simulink library "NMCCPG_Library"  (R2016b)
settings: Solver=VariableStepAuto  StartTime=0.0  StopTime=10.0  RelTol=1e-3  EnableMultiTasking=on
undefined symbols (not defined in the file or in its folder): CPG_On, CPGPhaseCheckTs, CPGSaved, N_record, N_start, NoiseFs, Pc, Var_Fm, Var_L, Var_Vel
libraries: simulink x4, dspsigops x4
settings Model: Creator=brug  LastModifiedBy=tycho
settings DataIOCC: LimitDataPoints=on
settings OptimizationCC: LifeSpan=inf
settings DebuggingCC: AllowSymbolicDim=off  SFUnexpectedBacktrackingDiag=warning  SFNoUnconditionalDefaultTransitionDiag=warning  SFExecutionAtInitializationDiag=none
settings ModelReferenceCC: PropagateSignalLabelsOutOfModel=off
settings GRTTargetCC: TargetLangStandard=C89/C90 (ANSI)
settings ConfigComp: CovMetricSettings=dw  CovHtmlReporting=on  CovSaveCumulativeToWorkspaceVar=on  CovSaveSingleToWorkspaceVar=on  CovExternalEMLEnable=off

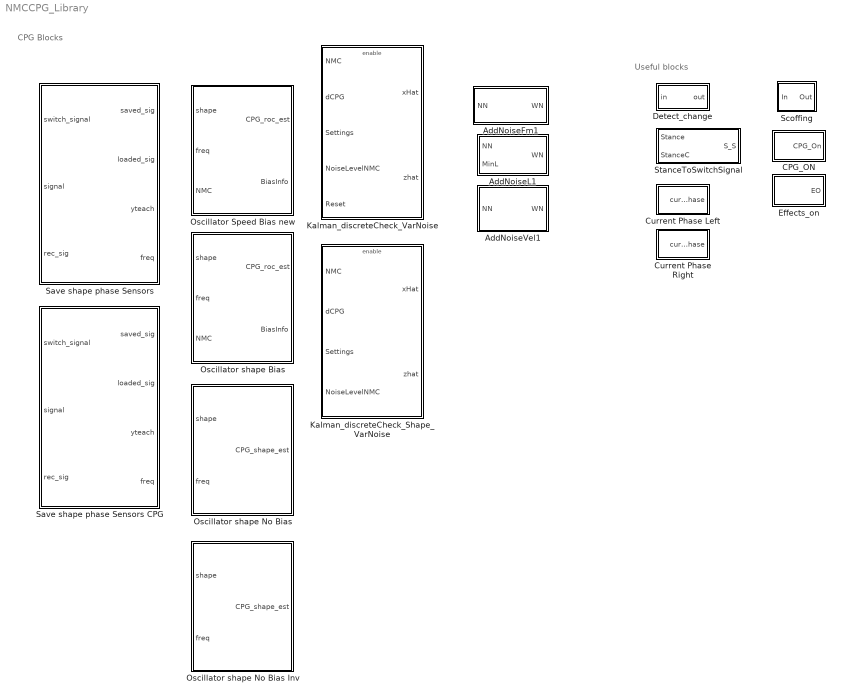
== system NMCCPG_Library ==
  note: CPG Blocks
  note: Useful blocks
  AddNoiseFm1 : Subsystem
  AddNoiseL1 : Subsystem
  AddNoiseVel1 : Subsystem
  CPG_ON : Subsystem
  Current Phase Left : Subsystem
  Current Phase Right : Subsystem
  Detect_change : Subsystem
  Effects_on : Subsystem
  Kalman_discreteCheck_Shape_VarNoise : Subsystem
      settings: MinAlgLoopOccurrences=on
  Kalman_discreteCheck_VarNoise : Subsystem
      settings: MinAlgLoopOccurrences=on
  "Oscillator Speed Bias new " : Subsystem
  Oscillator shape Bias : Subsystem
  Oscillator shape No Bias : Subsystem
  Oscillator shape No Bias Inv : Subsystem
  Save shape phase Sensors : Subsystem
  Save shape phase Sensors CPG : Subsystem
  Scoffing : Subsystem
  StanceToSwitchSignal : Subsystem

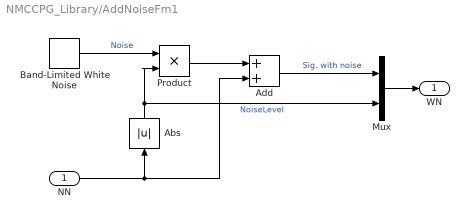
== system NMCCPG_Library/AddNoiseFm1 ==
  NN : Inport
  Abs : Abs
  Add : Sum
  Band-Limited White Noise : simulink/Sources/Band-Limited White Noise  Cov=[Var_Fm*(1/NoiseFs)]  Ts=(1/NoiseFs)  seed=[round(rand*10000)]
  Mux : Mux  Inputs=2
  Product : Product
  "WN " : Outport
  wires:
  Band-Limited White Noise/1 -> Product/1  "Noise"
  Product/1 -> Add/1
  NN/1 -> Abs/1, Add/2
  Add/1 -> Mux/1  "Sig. with noise"
  Mux/1 -> "WN "/1
  Abs/1 -> Product/2, Mux/2  "NoiseLevel"

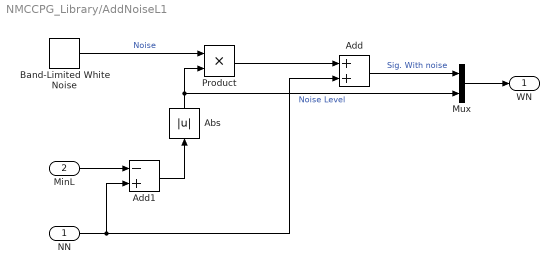
== system NMCCPG_Library/AddNoiseL1 ==
  NN : Inport
  MinL : Inport  Port=2
  Abs : Abs
  Add : Sum
  Add1 : Sum  Inputs=-+
  Band-Limited White Noise : simulink/Sources/Band-Limited White Noise  Cov=[Var_L*(1/NoiseFs)]  Ts=(1/NoiseFs)  seed=[round(rand*10000)]
  Mux : Mux  Inputs=2
  Product : Product
  "WN " : Outport
  wires:
  NN/1 -> Add1/2, Add/2
  Band-Limited White Noise/1 -> Product/1  "Noise"
  Product/1 -> Add/1
  Add1/1 -> Abs/1
  MinL/1 -> Add1/1
  Add/1 -> Mux/1  "Sig. With noise"
  Mux/1 -> "WN "/1
  Abs/1 -> Product/2, Mux/2  "Noise Level"

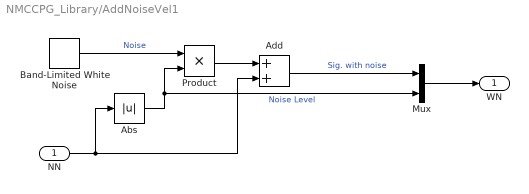
== system NMCCPG_Library/AddNoiseVel1 ==
  NN : Inport
  Abs : Abs
  Add : Sum
  Band-Limited White Noise : simulink/Sources/Band-Limited White Noise  Cov=[Var_Vel*(1/NoiseFs)]  Ts=(1/NoiseFs)  seed=[round(rand*10000)]
  Mux : Mux  Inputs=2
  Product : Product
  "WN " : Outport
  wires:
  NN/1 -> Add/2, Abs/1
  Abs/1 -> Mux/2, Product/2  "Noise Level"
  Band-Limited White Noise/1 -> Product/1  "Noise"
  Product/1 -> Add/1
  Mux/1 -> "WN "/1
  Add/1 -> Mux/1  "Sig. with noise"

== system NMCCPG_Library/CPG_ON ==
  Constant2 : Constant  Value=CPG_On
  Logical Operator : Logic  AllPortsSameDT=off  OutDataTypeStr=boolean
  CPG_On : Outport
  wires:
  [LR_saved_kept] -> Logical Operator/2
  Constant2/1 -> Logical Operator/1
  Logical Operator/1 -> CPG_On/1

== system NMCCPG_Library/Current Phase Left ==
  Sample and Hold3 : dspsigops/Sample and Hold  trig=Rising edge  initCond=0  latchinput=off
  cur_phase : Outport
  wires:
  Sample and Hold3/1 -> cur_phase/1
  [SwitchL] -> Sample and Hold3/Trigger, Sample and Hold3/1

== system NMCCPG_Library/Current Phase Right ==
  Sample and Hold3 : dspsigops/Sample and Hold  trig=Rising edge  initCond=0  latchinput=off
  cur_phase : Outport
  wires:
  [SwitchR] -> Sample and Hold3/1, Sample and Hold3/Trigger
  Sample and Hold3/1 -> cur_phase/1

== system NMCCPG_Library/Detect_change ==
  note: U(k)
  note: Edge
  in : Inport
  FixPt Relational Operator : RelationalOperator  Operator=~=  OutDataTypeStr=fixdt(0, 8)  ZeroCross=off  RndMeth=Nearest
  Memory : Memory
  "out " : Outport
  wires:
  Memory/1 -> FixPt Relational Operator/2  "U(k-1)"
  FixPt Relational Operator/1 -> "out "/1
  in/1 -> FixPt Relational Operator/1, Memory/1

== system NMCCPG_Library/Effects_on ==
  note: Used to turn on:
      | - Disturbances
      | - Noise on sensory signal
  Data Type Conversion : DataTypeConversion
  Transport Delay3 : TransportDelay  DelayTime=0.1
  EO : Outport
  wires:
  [LR_saved_kept] -> Data Type Conversion/1
  Transport Delay3/1 -> EO/1
  Data Type Conversion/1 -> Transport Delay3/1

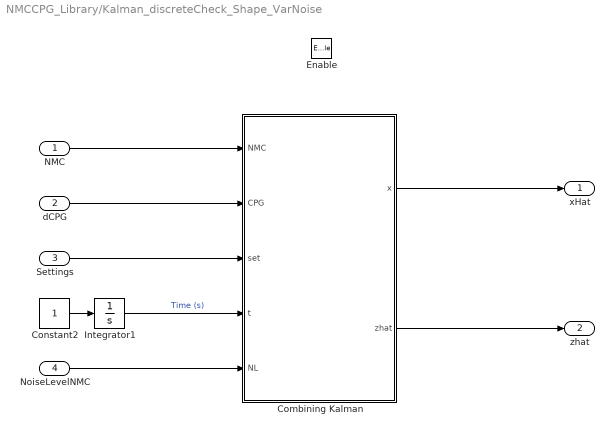
== system NMCCPG_Library/Kalman_discreteCheck_Shape_VarNoise ==
  NMC : Inport
  dCPG : Inport  Port=2
  Settings : Inport  Port=3
  NoiseLevelNMC : Inport  Port=4
  Enable : EnablePort  StatesWhenEnabling=reset
  Combining Kalman : MATLAB Function  SystemSampleTime=1E-3
      settings: MinAlgLoopOccurrences=on
  Constant2 : Constant
  Integrator1 : Integrator
  xHat : Outport
  zhat : Outport  Port=2
  wires:
  NoiseLevelNMC/1 -> Combining Kalman/5(NL)
  Combining Kalman/2(zhat) -> zhat/1
  Combining Kalman/1(x) -> xHat/1
  NMC/1 -> Combining Kalman/1(NMC)
  Settings/1 -> Combining Kalman/3(set)
  Constant2/1 -> Integrator1/1
  Integrator1/1 -> Combining Kalman/4(t)  "Time (s)"
  dCPG/1 -> Combining Kalman/2(CPG)

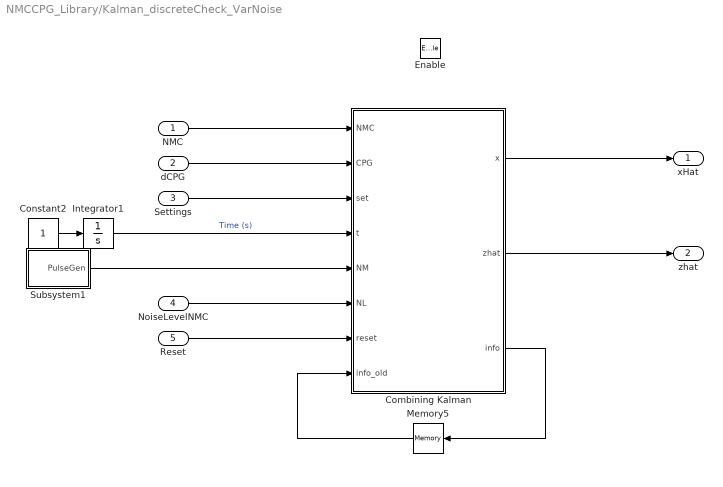
== system NMCCPG_Library/Kalman_discreteCheck_VarNoise ==
  NMC : Inport
  dCPG : Inport  Port=2
  Settings : Inport  Port=3
  NoiseLevelNMC : Inport  Port=4
  Reset : Inport  Port=5
  Enable : EnablePort  StatesWhenEnabling=reset
  Combining Kalman : MATLAB Function  TreatAsAtomicUnit=on  SystemSampleTime=1E-3
      settings: MinAlgLoopOccurrences=on
  Constant2 : Constant
  Integrator1 : Integrator
  Memory5 : Memory  X0=zeros(59,1)
  Subsystem1 : Subsystem
  xHat : Outport
  zhat : Outport  Port=2
  wires:
  Reset/1 -> Combining Kalman/7(reset)
  dCPG/1 -> Combining Kalman/2(CPG)
  Memory5/1 -> Combining Kalman/8(info_old)
  Combining Kalman/3(info) -> Memory5/1
  Integrator1/1 -> Combining Kalman/4(t)  "Time (s)"
  Constant2/1 -> Integrator1/1
  Subsystem1/1(PulseGen) -> Combining Kalman/5(NM)
  Settings/1 -> Combining Kalman/3(set)
  NMC/1 -> Combining Kalman/1(NMC)
  Combining Kalman/1(x) -> xHat/1
  Combining Kalman/2(zhat) -> zhat/1
  NoiseLevelNMC/1 -> Combining Kalman/6(NL)

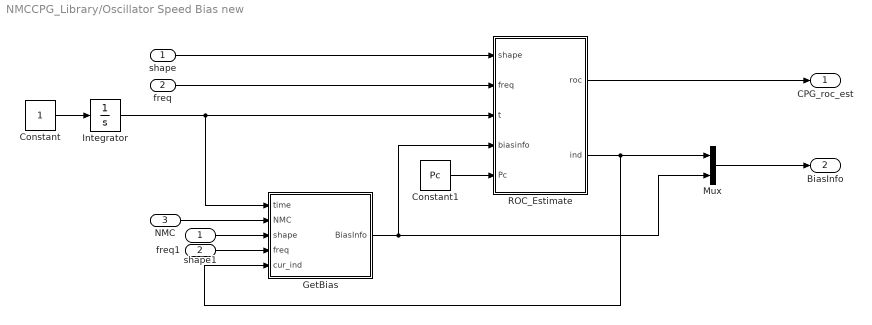
== system NMCCPG_Library/Oscillator Speed Bias new  ==
  shape : Inport
  freq : Inport  Port=2
  NMC : Inport  Port=3
  Constant : Constant
  Constant1 : Constant  Value=Pc
  GetBias : Subsystem
  Integrator : Integrator
  Mux : Mux  Inputs=2
  ROC_Estimate : MATLAB Function  TreatAsAtomicUnit=on
  freq1 : InportShadow  Port=2
  shape1 : InportShadow
  CPG_roc_est : Outport
  BiasInfo : Outport  Port=2
  wires:
  Constant1/1 -> ROC_Estimate/5(Pc)
  Mux/1 -> BiasInfo/1
  GetBias/1(BiasInfo) -> ROC_Estimate/4(biasinfo), Mux/2
  ROC_Estimate/2(ind) -> GetBias/5(cur_ind), Mux/1
  shape1/1 -> GetBias/3(shape)
  NMC/1 -> GetBias/2(NMC)
  Integrator/1 -> ROC_Estimate/3(t), GetBias/1(time)
  Constant/1 -> Integrator/1
  shape/1 -> ROC_Estimate/1(shape)
  ROC_Estimate/1(roc) -> CPG_roc_est/1
  freq/1 -> ROC_Estimate/2(freq)
  freq1/1 -> GetBias/4(freq)

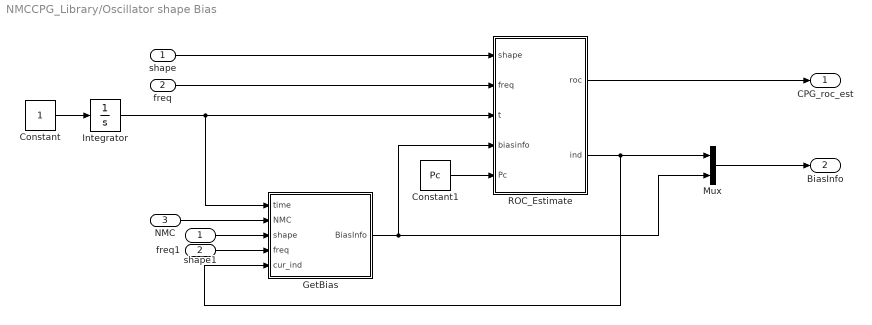
== system NMCCPG_Library/Oscillator shape Bias ==
  shape : Inport
  freq : Inport  Port=2
  NMC : Inport  Port=3
  Constant : Constant
  Constant1 : Constant  Value=Pc
  GetBias : Subsystem
  Integrator : Integrator
  Mux : Mux  Inputs=2
  ROC_Estimate : MATLAB Function  TreatAsAtomicUnit=on
  freq1 : InportShadow  Port=2
  shape1 : InportShadow
  CPG_roc_est : Outport
  BiasInfo : Outport  Port=2
  wires:
  freq1/1 -> GetBias/4(freq)
  freq/1 -> ROC_Estimate/2(freq)
  ROC_Estimate/1(roc) -> CPG_roc_est/1
  shape/1 -> ROC_Estimate/1(shape)
  Constant/1 -> Integrator/1
  Integrator/1 -> GetBias/1(time), ROC_Estimate/3(t)
  NMC/1 -> GetBias/2(NMC)
  shape1/1 -> GetBias/3(shape)
  ROC_Estimate/2(ind) -> Mux/1, GetBias/5(cur_ind)
  GetBias/1(BiasInfo) -> Mux/2, ROC_Estimate/4(biasinfo)
  Mux/1 -> BiasInfo/1
  Constant1/1 -> ROC_Estimate/5(Pc)

== system NMCCPG_Library/Oscillator shape No Bias ==
  shape : Inport
  freq : Inport  Port=2
  Constant : Constant
  Integrator : Integrator
  ROC_Estimate : MATLAB Function  TreatAsAtomicUnit=on  SystemSampleTime=1e-2
      settings: MinAlgLoopOccurrences=on
  CPG_shape_est : Outport
  wires:
  freq/1 -> ROC_Estimate/2(freq)
  ROC_Estimate/1(cpg_out) -> CPG_shape_est/1
  shape/1 -> ROC_Estimate/1(shape)
  Constant/1 -> Integrator/1
  Integrator/1 -> ROC_Estimate/3(t)

== system NMCCPG_Library/Oscillator shape No Bias Inv ==
  shape : Inport
  freq : Inport  Port=2
  Constant : Constant
  Integrator : Integrator
  ROC_Estimate : MATLAB Function  TreatAsAtomicUnit=on
      settings: MinAlgLoopOccurrences=on
  CPG_shape_est : Outport
  wires:
  Integrator/1 -> ROC_Estimate/3(t)
  Constant/1 -> Integrator/1
  shape/1 -> ROC_Estimate/1(shape)
  ROC_Estimate/1(cpg_out) -> CPG_shape_est/1
  freq/1 -> ROC_Estimate/2(freq)

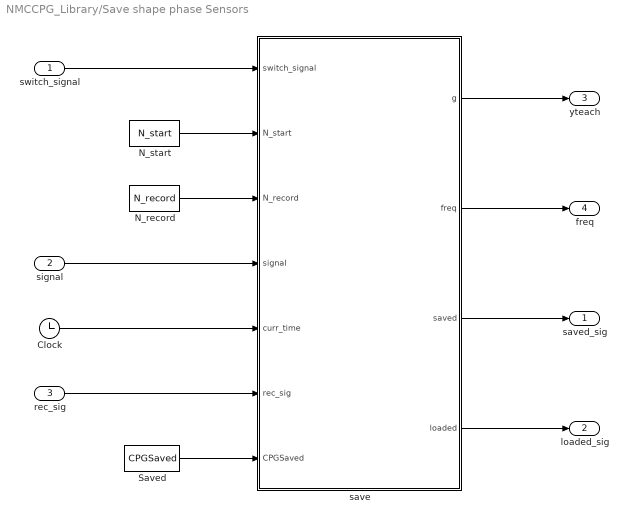
== system NMCCPG_Library/Save shape phase Sensors ==
  switch_signal : Inport
  signal : Inport  Port=2
  rec_sig : Inport  Port=3
  Clock : Clock
      settings: Decimation=1E6
  N_record : Constant  Value=N_record
  N_start : Constant  Value=N_start
  Saved : Constant  Value=CPGSaved
  save : Stateflow chart  TreatAsAtomicUnit=on
  saved_sig : Outport
  loaded_sig : Outport  Port=2
  yteach : Outport  Port=3
  freq : Outport  Port=4
  wires:
  Saved/1 -> save/7(CPGSaved)
  switch_signal/1 -> save/1(switch_signal)
  N_record/1 -> save/3(N_record)
  signal/1 -> save/4(signal)
  save/2(freq) -> freq/1
  N_start/1 -> save/2(N_start)
  save/1(g) -> yteach/1
  save/3(saved) -> saved_sig/1
  Clock/1 -> save/5(curr_time)
  rec_sig/1 -> save/6(rec_sig)
  save/4(loaded) -> loaded_sig/1

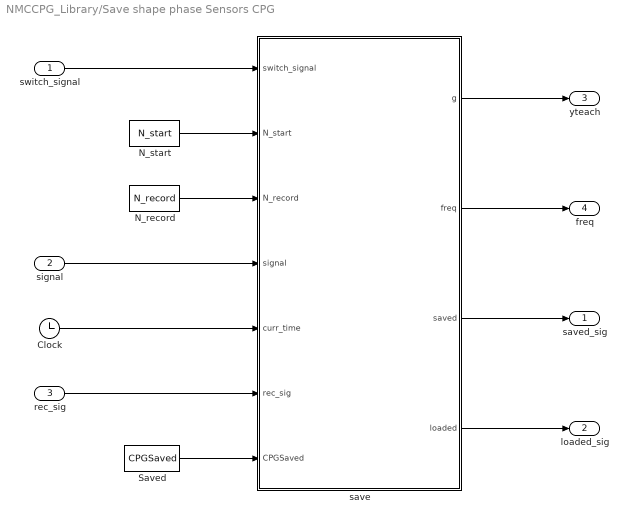
== system NMCCPG_Library/Save shape phase Sensors CPG ==
  switch_signal : Inport
  signal : Inport  Port=2
  rec_sig : Inport  Port=3
  Clock : Clock
      settings: Decimation=1E6
  N_record : Constant  Value=N_record
  N_start : Constant  Value=N_start
  Saved : Constant  Value=CPGSaved
  save : Stateflow chart  TreatAsAtomicUnit=on
  saved_sig : Outport
  loaded_sig : Outport  Port=2
  yteach : Outport  Port=3
  freq : Outport  Port=4
  wires:
  save/4(loaded) -> loaded_sig/1
  rec_sig/1 -> save/6(rec_sig)
  Clock/1 -> save/5(curr_time)
  save/3(saved) -> saved_sig/1
  save/1(g) -> yteach/1
  N_start/1 -> save/2(N_start)
  save/2(freq) -> freq/1
  signal/1 -> save/4(signal)
  N_record/1 -> save/3(N_record)
  switch_signal/1 -> save/1(switch_signal)
  Saved/1 -> save/7(CPGSaved)

== system NMCCPG_Library/Scoffing ==
  note: This Block keeps the swing phase active for 0.1s in case of scoffing
  In : Inport
  Compare To Zero : simulink/Logic and Bit Operations/Compare To Zero  relop=>  OutDataTypeStr=boolean
  Data Type Conversion : DataTypeConversion
  Logical Operator : Logic  Operator=OR  AllPortsSameDT=off  OutDataTypeStr=boolean
  Transport Delay : TransportDelay  DelayTime=0.1
  Out : Outport
  wires:
  Transport Delay/1 -> Compare To Zero/1
  In/1 -> Data Type Conversion/1, Logical Operator/2
  Logical Operator/1 -> Out/1
  Data Type Conversion/1 -> Transport Delay/1
  Compare To Zero/1 -> Logical Operator/1

== system NMCCPG_Library/StanceToSwitchSignal ==
  note: Change signal:
      | 1 - Stance
      | 2 - Swing
  Stance : Inport
  StanceC : Inport  Port=2
  MATLAB Function : MATLAB Function  TreatAsAtomicUnit=on
  S_S : Outport
  wires:
  StanceC/1 -> MATLAB Function/2(u2)
  MATLAB Function/1(y) -> S_S/1
  Stance/1 -> MATLAB Function/1(u1)

== system NMCCPG_Library/Kalman_discreteCheck_VarNoise/Subsystem1 ==
  Abs : Abs
  Add : Sum  Inputs=+-
  Memory : Memory
  Pulse Generator : DiscretePulseGenerator  PulseType=Time based  Period=(1/NoiseFs)*2  PulseWidth=50  SampleTime=-1
  PulseGen : Outport
  wires:
  Add/1 -> Abs/1
  Abs/1 -> PulseGen/1
  Memory/1 -> Add/2
  Pulse Generator/1 -> Add/1, Memory/1

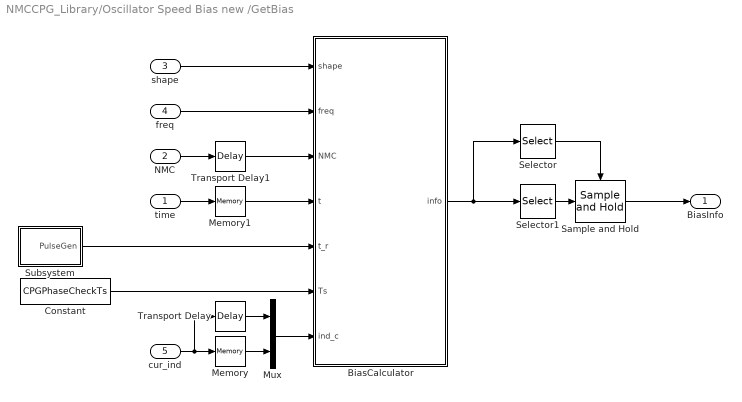
== system NMCCPG_Library/Oscillator Speed Bias new /GetBias ==
  time : Inport
  NMC : Inport  Port=2
  shape : Inport  Port=3
  freq : Inport  Port=4
  cur_ind : Inport  Port=5
  BiasCalculator : MATLAB Function  TreatAsAtomicUnit=on
  Constant : Constant  Value=CPGPhaseCheckTs
  Memory : Memory
  Memory1 : Memory
  Mux : Mux  Inputs=2
  Sample and Hold : dspsigops/Sample and Hold  trig=Rising edge  initCond=[]  latchinput=off
  Selector : Selector  InputPortWidth=4  IndexOptions=Index vector (dialog)  Indices=[1]  OutputSizes=1
  Selector1 : Selector  InputPortWidth=4  IndexOptions=Index vector (dialog)  Indices=[2:4]  OutputSizes=1
  Subsystem : Subsystem
  Transport Delay : TransportDelay  DelayTime=CPGPhaseCheckTs*0.5
  Transport Delay1 : TransportDelay  DelayTime=CPGPhaseCheckTs*0.5  InitialOutput=zeros(19,1)
  BiasInfo : Outport
  wires:
  Transport Delay1/1 -> BiasCalculator/3(NMC)
  Selector1/1 -> Sample and Hold/1
  Memory1/1 -> BiasCalculator/4(t)
  Mux/1 -> BiasCalculator/7(ind_c)
  Transport Delay/1 -> Mux/1
  Memory/1 -> Mux/2
  Selector/1 -> Sample and Hold/Trigger
  Sample and Hold/1 -> BiasInfo/1
  Subsystem/1(PulseGen) -> BiasCalculator/5(t_r)
  Constant/1 -> BiasCalculator/6(Ts)
  shape/1 -> BiasCalculator/1(shape)
  BiasCalculator/1(info) -> Selector/1, Selector1/1
  cur_ind/1 -> Memory/1, Transport Delay/1
  time/1 -> Memory1/1
  NMC/1 -> Transport Delay1/1
  freq/1 -> BiasCalculator/2(freq)

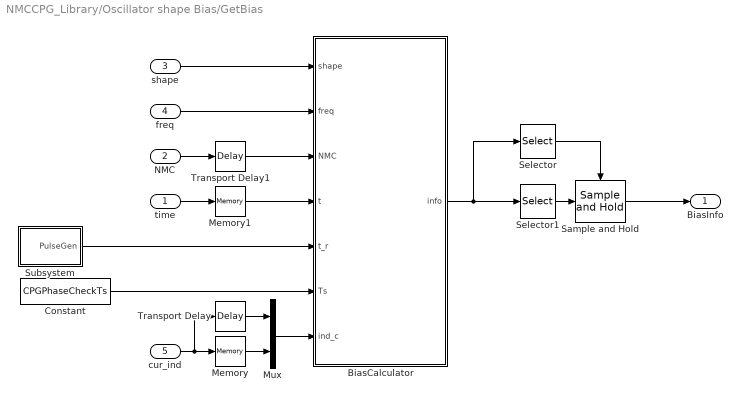
== system NMCCPG_Library/Oscillator shape Bias/GetBias ==
  time : Inport
  NMC : Inport  Port=2
  shape : Inport  Port=3
  freq : Inport  Port=4
  cur_ind : Inport  Port=5
  BiasCalculator : MATLAB Function  TreatAsAtomicUnit=on
  Constant : Constant  Value=CPGPhaseCheckTs
  Memory : Memory
  Memory1 : Memory
  Mux : Mux  Inputs=2
  Sample and Hold : dspsigops/Sample and Hold  trig=Rising edge  initCond=[]  latchinput=off
  Selector : Selector  InputPortWidth=4  IndexOptions=Index vector (dialog)  Indices=[1]  OutputSizes=1
  Selector1 : Selector  InputPortWidth=4  IndexOptions=Index vector (dialog)  Indices=[2:4]  OutputSizes=1
  Subsystem : Subsystem
  Transport Delay : TransportDelay  DelayTime=CPGPhaseCheckTs*0.5
  Transport Delay1 : TransportDelay  DelayTime=CPGPhaseCheckTs*0.5  InitialOutput=zeros(19,1)
  BiasInfo : Outport
  wires:
  freq/1 -> BiasCalculator/2(freq)
  NMC/1 -> Transport Delay1/1
  time/1 -> Memory1/1
  cur_ind/1 -> Transport Delay/1, Memory/1
  BiasCalculator/1(info) -> Selector1/1, Selector/1
  shape/1 -> BiasCalculator/1(shape)
  Constant/1 -> BiasCalculator/6(Ts)
  Subsystem/1(PulseGen) -> BiasCalculator/5(t_r)
  Sample and Hold/1 -> BiasInfo/1
  Selector/1 -> Sample and Hold/Trigger
  Memory/1 -> Mux/2
  Transport Delay/1 -> Mux/1
  Mux/1 -> BiasCalculator/7(ind_c)
  Memory1/1 -> BiasCalculator/4(t)
  Selector1/1 -> Sample and Hold/1
  Transport Delay1/1 -> BiasCalculator/3(NMC)

== system NMCCPG_Library/Oscillator Speed Bias new /GetBias/Subsystem ==
  note: PulseGen outputs a 1 every after every CPGPhaseCheckTs (s)
  Abs : Abs
  Add : Sum  Inputs=+-
  Memory : Memory
  Pulse Generator : DiscretePulseGenerator  PulseType=Time based  Period=CPGPhaseCheckTs*2  PulseWidth=50  SampleTime=-1
  PulseGen : Outport
  wires:
  Add/1 -> Abs/1
  Abs/1 -> PulseGen/1
  Memory/1 -> Add/2
  Pulse Generator/1 -> Add/1, Memory/1

== system NMCCPG_Library/Oscillator shape Bias/GetBias/Subsystem ==
  note: PulseGen outputs a 1 every after every CPGPhaseCheckTs (s)
  Abs : Abs
  Add : Sum  Inputs=+-
  Memory : Memory
  Pulse Generator : DiscretePulseGenerator  PulseType=Time based  Period=CPGPhaseCheckTs*2  PulseWidth=50  SampleTime=-1
  PulseGen : Outport
  wires:
  Pulse Generator/1 -> Memory/1, Add/1
  Memory/1 -> Add/2
  Abs/1 -> PulseGen/1
  Add/1 -> Abs/1

== matlab function NMCCPG_Library/Oscillator Speed Bias new /GetBias/BiasCalculator ==
  data: shape input; freq input; NMC input; t input; t_r input; Ts input; ind_c input; info output
function info  = fcn(shape,freq,NMC,t,t_r,Ts,ind_c)
%% SizeSettings
N = size(shape,2);
p_area = Ts*freq;

%% Initial conditions
if t < Ts
    info = [2+t;0;1;0];
else
    if t_r == 1 
        %% Estimated indices
        fg = ind_c(1);
        
        %% Setting size
        assert(fg<N*2) 
        assert(fg>-N*2);
        assert(p_area<10) 
        assert(p_area>-1);
        
        %% Max area
        area = round(fg)-round(p_area*N):round(fg)+round(p_area*N);
        area(area<1) = [];area(area>N) = [];
        
        %% Finding optimal index in shape
        cur = repmat(NMC,1,length(area));
        [~,ind2] = min(sum(abs(shape(:,area)-cur)));
        ind = ind2 + min(area) - 1;
        
        %% Calculating Bias
        bias = ind - fg;
        
        %% Setting output
        info = [1;bias;ind_c(2);t];
    else
        %% BiasCheck is only active if t_r == 1
        info = zeros(4,1);
    end
end

== matlab function NMCCPG_Library/Oscillator Speed Bias new /ROC_Estimate ==
  data: shape input; roc output; freq input; t input; biasinfo input; ind output; Pc input
function [roc,ind] = roc_est(shape,freq,t,biasinfo,Pc)
%% Pre-allocating
N = size(shape,2);
M = size(shape,1);
roc = zeros(M,1);

%% Estimating current indices in Shape
% Initial conditions
if t < 0.05 || biasinfo(2,1) == 1
    biasinfo = [0;1;0];
end

%% Calculating frequency
freq_n = (biasinfo(1,1)/(Pc*(N-1)))+freq;

%% Estimating current index in shape
ind = biasinfo(2,1) + (N-1)*(t-biasinfo(3,1))*freq_n;

%% Flooring and finding diff
ind_fl = floor(ind);
int_diff = ind-ind_fl;

%% Setting bounds
if ind > N
    ind = N;
    ind_fl = N;
end
assert(ind_fl<N+1) 
assert(ind_fl>0);

%% Calculating speed using 9 point diff and interpolating for extra accuracy
ind_l = zeros(1,10);
ind_l(1,:) = ind_fl-4:ind_fl+5;
if ind_l(1) >= 1 && ind_l(end) <= N
    x_int = zeros(M,9);
    x_int(:,:) = interp1(ind_l,shape(:,ind_l)',ind_l(1:end-1)+int_diff)';
    speed = sum(x_int.*repmat([1/280 -4/105 1/5 -4/5 0 4/5 -1/5 4/105 -1/280]*((N-1)*freq),size(x_int,1),1),2);
elseif ind_l(1) < 1
    x_int = zeros(M,5);
    x_int(:,:) = interp1(ind_l(5:end),shape(:,ind_l(5:end))',ind_l(5:end-1)+int_diff)';
    speed = sum(x_int.*repmat([-25/12 4 -3 4/3 -1/4]*((N-1)*freq),size(x_int,1),1),2);
elseif ind_l(6) < N
    x_int = zeros(M,5);
    x_int(:,:) = interp1(ind_l(1:6),shape(:,ind_l(1:6))',ind_l(1:5)+int_diff)';
    speed = sum(x_int.*repmat([1/4 -4/3 3 -4 25/12]*((N-1)*freq),size(x_int,1),1),2);
else
    speed = sum(shape(:,end-4:end).*repmat([1/4 -4/3 3 -4 25/12]*((N-1)*freq),size(shape(:,end-4:end),1),1),2);
end 

%% Output
roc(:,1) = speed;
end

== matlab function NMCCPG_Library/Oscillator shape Bias/GetBias/BiasCalculator ==
  data: shape input; freq input; NMC input; t input; t_r input; Ts input; ind_c input; info output
function info  = fcn(shape,freq,NMC,t,t_r,Ts,ind_c)
%% SizeSettings
N = size(shape,2);
p_area = Ts*freq;

%% Initial conditions
if t < Ts
    info = [2+t;0;1;0];
else
    if t_r == 1 
        %% Estimated indices
        fg = ind_c(1);
        
        %% Setting size
        assert(fg<N*2) 
        assert(fg>-N*2);
        assert(p_area<10) 
        assert(p_area>-1);
        
        %% Max area
        area = round(fg)-round(p_area*N):round(fg)+round(p_area*N);
        area(area<1) = [];area(area>N) = [];
        
        %% Finding optimal index in shape
        cur = repmat(NMC,1,length(area));
        [~,ind2] = min(sum(abs(shape(:,area)-cur)));
        ind = ind2 + min(area) - 1;
        
        %% Calculating Bias
        bias = ind - fg;
        
        %% Setting output
        info = [1;bias;ind_c(2);t];
    else
        %% BiasCheck is only active if t_r == 1
        info = zeros(4,1);
    end
end

== matlab function NMCCPG_Library/Oscillator shape Bias/ROC_Estimate ==
  data: shape input; roc output; freq input; t input; biasinfo input; ind output; Pc input
function [roc,ind] = roc_est(shape,freq,t,biasinfo,Pc)
%% Pre-allocating
N = size(shape,2);
M = size(shape,1);
roc = zeros(M,1);

%% Estimating current indices in Shape
% Initial conditions
if t < 0.05 || biasinfo(2,1) == 1
    biasinfo = [0;1;0];
end

%% Calculating frequency
freq_n = (biasinfo(1,1)/(Pc*(N-1)))+freq;

%% Estimating current index in shape
ind = biasinfo(2,1) + (N-1)*(t-biasinfo(3,1))*freq_n;

%% Flooring and finding diff
ind_fl = floor(ind);
int_diff = ind-ind_fl;

%% Setting bounds
if ind > N
    ind = N;
    ind_fl = N;
end
assert(ind_fl<N+1) 
assert(ind_fl>0);

%% Calculating speed using 9 point diff and interpolating for extra accuracy
ind_l = zeros(1,2);
ind_l(1,:) = ind_fl:ind_fl+1;
if ind_l(end) <= N
    speed = zeros(M,1);
    speed(:,1) = interp1(ind_l,shape(:,ind_l)',ind_l(1)+int_diff)';
else
    speed = shape(:,N);
end 

%% Output
roc(:,1) = speed;
end

== matlab function NMCCPG_Library/Kalman_discreteCheck_Shape_VarNoise/Combining Kalman ==
  data: NMC input; CPG input; set input; t input; NL input; x output; zhat output
function [x,zhat]  = fcn(NMC,CPG,set,t,NL)
%% Predefining
x = zeros(19,1);
zhat = zeros(19,1);

if t < 0.1
    %% Initialisation
    x(:,1) = NMC;
    zhat = NMC;
else
    %%KALMAN
    %% Defining param
    Cw = diag(set(:,2));
    Cn = diag(set(:,1).*(NL.^2));
    
    %% A Priori
    x_2_1 = CPG;
    zhat(:,1) = x_2_1;
    
    %% A posteriori in case of measurement
    S = Cw + Cn;
    K = (Cw)/(S);
    x_2_2 = x_2_1 + K * (NMC-zhat);
    
    x(:,1) = x_2_2;
end
end

== matlab function NMCCPG_Library/Oscillator shape No Bias Inv/ROC_Estimate ==
  data: shape input; cpg_out output; freq input; t input
function cpg_out  = roc_est(shape,freq,t)
%% Pre-allocating
N = size(shape,2);
M = size(shape,1);
cpg_out = zeros(M,1);

%% Estimating current indices in Shape
%% Estimating current index in shape
ind = 1 + (N-1)*(t)*freq;

%% Flooring and finding diff
ind_fl = floor(ind);
int_diff = ind-ind_fl;

%% Setting bounds
if ind > N
    ind = N;
    ind_fl = N;
end
assert(ind_fl<N+1) 
assert(ind_fl>0);

%% Calculating Estimated point
ind_l = zeros(1,2);
ind_l(1,:) = ind_fl:ind_fl+1;
if ind_l(end) <= N
    est = zeros(M,1);
    est(:,1) = interp1(ind_l,shape(:,ind_l)',ind_l(1)+int_diff)';
else
    est = shape(:,N);
end 

%% Output
cpg_out(:,1) = est;
end

== matlab function NMCCPG_Library/StanceToSwitchSignal/MATLAB Function ==
  data: u1 input; y output; u2 input
function y = fcn(u1, u2)
if u1 == 1 && u2 == 1
    y = 1;
elseif u1 == 0 && u2 == 1
    y = 2;
else 
    y = 0;
end

== stateflow chart NMCCPG_Library/Save shape phase Sensors/save ==
  state START
    entry:
    saved=0;
    number_of_switch=0;
    g = zeros(1,CPGSize);
    signal_recorded=0;tc=0;mean_sectemp =0;
    during:
    if (switch_signal==rec_sig)
    number_of_switch=number_of_switch+1;
    end
  state RECORD
    entry:
    B = ones(1,1E4);
    Btime = ones(1,1E4)*1E5;
    i=1;i2 = 1;
    during:
    if switch_signal ~= 0 &&switch_signal~=rec_sig
    i2 = 2;
    end
    if i2 == 1
    B(:,i) = signal;
    Btime(i) = curr_time;
    i=i+1;
    end
    exit:
    if(switch_signal==rec_sig && signal_recorded<N_record)
    signal_recorded=signal_recorded+1;
    [C,tc]=interpolate_cpg(B,Btime,CPGSize);
    g = g*((signal_recorded-1)/signal_recorded) +C*(1/signal_recorded);
    mean_sectemp =mean_sectemp*((signal_recorded-1)/signal_recorded)+tc*(1/signal_recorded);
    freq = 1./mean_sectemp;
    end
  state Load
    entry:
    loaded = 1;
  state SAVE
    entry:
    saved = 1;
  state END
    entry:
    saved = 0;
    loaded = 0;
  (default) -> START
  START -> Load [order 2] : [(switch_signal==rec_sig && number_of_switch == N_start&&CPGSaved == 1)||(CPGSaved == 1&&N_start==0)]
  START -> RECORD [order 1] : [switch_signal==rec_sig && number_of_switch == N_start&&CPGSaved == 0]
  Load -> END : [loaded==1]
  RECORD -> RECORD [order 1] : [switch_signal==rec_sig && signal_recorded<N_record]
  RECORD -> SAVE [order 2] : [signal_recorded==N_record]
  SAVE -> END : [saved == 1]
  data: x function_input; X function_output; t_dur function_output; xtime function_input; size function_input; switch_signal input; N_start input; N_record input; signal_recorded local size=1; number_of_switch local; signal input; i local size=1; B local size=[1,1E4]; C local size=[1,CPGSize]; g output size=[1,CPGSize]; freq output; mean_sectemp local; saved output size=1; curr_time input; Btime local size=[1,1E4]; i2 local size=1; tc local; rec_sig input; CPGSaved input; loaded output; CPGSize constant double =CPGSize
  function [X,t_dur]=interpolate_cpg(x,xtime,size):
    | function [X,t_dur]=interpolate_cpg(x,xtime,size)
    | X_sav = zeros(1,size);
    | 
    | fc = find(xtime~=1E5);
    | 
    | t_temp=xtime(fc);
    | x_temp=x(:,fc);
    | x_temp = x_temp';
    | 
    | t_dur = t_temp(end)-t_temp(1);
    | 
    | X_sav(:,:)=interp1(t_temp,x_temp,linspace(t_temp(1),t_temp(end),size))';
    | X=X_sav;
    | end

== stateflow chart NMCCPG_Library/Save shape phase Sensors CPG/save ==
  state START
    entry:
    saved=0;
    number_of_switch=0;
    g = zeros(1,CPGSize);
    signal_recorded=0;tc=0;mean_sectemp =0;
    during:
    if (switch_signal==rec_sig)
    number_of_switch=number_of_switch+1;
    end
  state RECORD
    entry:
    B = ones(1,1E4);
    Btime = ones(1,1E4)*1E5;
    i=1;i2 = 1;
    during:
    if switch_signal ~= 0 &&switch_signal~=rec_sig
    i2 = 2;
    if i ~= 1
    signal_recorded=signal_recorded+1;
    [C,tc]=interpolate_cpg(B,Btime,CPGSize);
    g = g*((signal_recorded-1)/signal_recorded) +C*(1/signal_recorded);
    mean_sectemp =mean_sectemp*((signal_recorded-1)/signal_recorded)+tc*(1/signal_recorded);
    freq = 1./mean_sectemp;
    i = 1;
    end
    end
    if i2 == 1
    B(:,i) = signal;
    Btime(i) = curr_time;
    i=i+1;
    end
  state Load
    entry:
    loaded = 1;
  state SAVE
    entry:
    saved = 1;
  state END
    entry:
    saved = 0;
    loaded = 0;
  (default) -> START
  START -> Load [order 2] : [(switch_signal==rec_sig && number_of_switch == N_start&&CPGSaved == 1)||(CPGSaved == 1&&N_start==0)]
  START -> RECORD [order 1] : [switch_signal==rec_sig && number_of_switch == N_start&&CPGSaved == 0]
  Load -> END : [loaded==1]
  RECORD -> RECORD [order 1] : [switch_signal==rec_sig && signal_recorded<N_record]
  RECORD -> SAVE [order 2] : [signal_recorded==N_record]
  SAVE -> END : [saved == 1]
  data: x function_input; X function_output; t_dur function_output; xtime function_input; size function_input; switch_signal input; N_start input; N_record input; signal_recorded local size=1; number_of_switch local; signal input; i local size=1; B local size=[1,1E4]; C local size=[1,CPGSize]; g output size=[1,CPGSize]; freq output; mean_sectemp local; saved output size=1; curr_time input; Btime local size=[1,1E4]; i2 local size=1; tc local; rec_sig input; CPGSaved input; loaded output; CPGSize constant double =CPGSize
  function [X,t_dur]=interpolate_cpg(x,xtime,size):
    | function [X,t_dur]=interpolate_cpg(x,xtime,size)
    | X_sav = zeros(1,size);
    | 
    | fc = find(xtime~=1E5);
    | 
    | t_temp=xtime(fc);
    | x_temp=x(:,fc);
    | x_temp = x_temp';
    | 
    | t_dur = t_temp(end)-t_temp(1);
    | 
    | X_sav(:,:)=interp1(t_temp,x_temp,linspace(t_temp(1),t_temp(end),size))';
    | X=X_sav;
    | end

== matlab function NMCCPG_Library/Oscillator shape No Bias/ROC_Estimate ==
  data: shape input; cpg_out output; freq input; t input
function cpg_out  = roc_est(shape,freq,t)
%% Pre-allocating
N = size(shape,2);
M = size(shape,1);
cpg_out = zeros(M,1);

%% Estimating current indices in Shape
%% Estimating current index in shape
ind = 1 + (N-1)*(t)*freq;

%% Flooring and finding diff
ind_fl = floor(ind);
int_diff = ind-ind_fl;

%% Setting bounds
if ind > N
    ind = N;
    ind_fl = N;
end
assert(ind_fl<N+1) 
assert(ind_fl>0);

%% Calculating Estimated point
ind_l = zeros(1,2);
ind_l(1,:) = ind_fl:ind_fl+1;
if ind_l(end) <= N
    est = zeros(M,1);
    est(:,1) = interp1(ind_l,shape(:,ind_l)',ind_l(1)+int_diff)';
else
    est = shape(:,N);
end 

%% Output
cpg_out(:,1) = est;
end

== matlab function NMCCPG_Library/Kalman_discreteCheck_VarNoise/Combining Kalman ==
  data: NMC input; CPG input; set input; t input; NM input; NL input; reset input; info_old input; x output; zhat output; info output
function [x,zhat,info]  = fcn(NMC,CPG,set,t,NM,NL,reset,info_old)
%% Loading data
x_old = info_old(1:19,1);
C_old = info_old(20:38,1);
CPG_old = info_old(39:57,1);
t_old = info_old(end-1,1);
phase_old = info_old(end,1);

%% Predefining
x = zeros(19,1);
zhat = zeros(19,1);
info = zeros(59,1);

%% Params
dt = (t-t_old);
B = dt*eye(19);
dCPG_out = CPG; 
t_out = t;

if t < 0.1
    %% Initialisation
    x(:,1) = NMC;
    C = zeros(19,1);
    zhat = NMC;
else
    %%KALMAN
    %% Defining param
    C_1_1 = diag(C_old);   
    Cw = diag(set(:,2));   
    Cn = diag(set(:,1).*(NL.^2));   
    u_1_1 = CPG_old;
    
    %% A Priori
    x_2_1 = x_old + B * u_1_1;
    C_2_1 = C_1_1 + B*Cw;
    zhat(:,1) = x_2_1;
    
    if NM == 1
        %% A posteriori in case of measurement
        S = C_2_1 + Cn;
        K = (C_2_1)/(S);
        x_2_2 = x_2_1 + K * (NMC-zhat);
        D = (eye(19)-K);
        C_2_2 = D*C_2_1*D' + K*Cn*K';

        x(:,1) = x_2_2;
        C = C_2_2*ones(size(C_2_2,2),1);
    else
        %% A posteriori in case of no new measurement
        x(:,1) = x_2_1;
        C = C_2_1*ones(size(C_2_1,2),1);
    end
end
info(:,1) = [x;C;dCPG_out;t_out;reset(end)];

%% Reset after event
if (phase_old ~= reset(end)) && reset(end) == 1
    info(1:19,1) = reset(1:19,1);
elseif (phase_old ~= reset(end)) && reset(end) == 2
    info(1:19,1) = reset(20:38,1);
end
end
